simulink model "EKF_SIL_02_newdelIps"  (R2015a)
settings: Solver=ode45  StartTime=0.0  StopTime=totalSimulationTime  RelTol=1e-3
model workspace: external: MATLAB File Init_Model_02_Simulink_SIL1.m (data not in the file)
values from neighbouring files (symbols this model uses):
  Cov_nu = [0.005 0 0 0 ... (first row only)    [InitOOSM.m]    (also in InitSIL.m; Init_Model_02_Simulink.m; Init_Model_02_Simulink_SIL1.m)
  Cov_r = [0.003 0 0 ... (first row only)    [InitOOSM.m]    (also in InitSIL.m; Init_Model_02_Simulink.m; Init_Model_02_Simulink_SIL1.m)
  e_force_x = 0    [InitOOSM.m]    (also in InitSIL.m; Init_Model_02_Simulink.m; Init_Model_02_Simulink_SIL1.m)
  e_force_y = 0    [InitOOSM.m]    (also in InitSIL.m; Init_Model_02_Simulink.m; Init_Model_02_Simulink_SIL1.m)
  e_force_z = 0    [InitOOSM.m]    (also in InitSIL.m; Init_Model_02_Simulink.m; Init_Model_02_Simulink_SIL1.m)
  ieps = [-0.7071;0;0;0.7071]    [InitOOSM.m]    (also in InitSIL.m; Init_Model_02_Simulink.m = [-0.7071; 0; 0; 0.7071]; Init_Model_02_Simulink_SIL1.m)
  ita = [0.5;0.5;0.5;0.5]    [InitOOSM.m]    (also in InitSIL.m; Init_Model_02_Simulink.m = [0.5; 0.5; 0.5; 0.5]; Init_Model_02_Simulink_SIL1.m)
  n = 0.00    (= 0)    [InitOOSM.m]    (also in InitSIL.m; Init_Model_02_Simulink.m; Init_Model_02_Simulink_SIL1.m)
  P_0 = 0.5*eye(18,18)    [InitOOSM.m]    (also in InitSIL.m = 0.05*eye(12,12); Init_Model_02_Simulink.m = 0.005*eye(12,12); Init_Model_02_Simulink_SIL1.m = 0.005*eye(12,12))
  p_x = 0.75    [InitOOSM.m]    (also in InitSIL.m; Init_Model_02_Simulink.m; Init_Model_02_Simulink_SIL1.m)
  p_y = 0.125    [InitOOSM.m]    (also in InitSIL.m; Init_Model_02_Simulink.m; Init_Model_02_Simulink_SIL1.m)
  p_z = -0.8    [InitOOSM.m]    (also in InitSIL.m; Init_Model_02_Simulink.m; Init_Model_02_Simulink_SIL1.m)
  parameter_gravitation = 3.986005E+14    (= 398600500000000)    [InitOOSM.m]    (also in InitSIL.m; Init_Model_02_Simulink.m; Init_Model_02_Simulink_SIL1.m)
  rho = [0.04;0;0.3]    [InitOOSM.m]    (also in InitSIL.m; Init_Model_02_Simulink.m = [0.04; 0; 0.3]; Init_Model_02_Simulink_SIL1.m)
  rho_c = [-0.00017;   -0.9780;   -0.1854]    [InitOOSM.m]    (also in InitSIL.m = [0.00036;   -0.9865;   -0.1854]; Init_Model_02_Simulink.m = [0.00036; -0.9865; -0.1854]; Init_Model_02_Simulink_SIL1.m = [0.00036;   -0.9865;   -0.1854])
  sig_f = 2E-6    (= 2e-06)    [InitOOSM.m]    (also in InitSIL.m; Init_Model_02_Simulink.m; Init_Model_02_Simulink_SIL1.m)
  sig_tau = 2.5E-5    (= 2.5e-05)    [InitOOSM.m]    (also in InitSIL.m; Init_Model_02_Simulink.m; Init_Model_02_Simulink_SIL1.m)
  t_delta = 0.2    [InitOOSM.m]    (also in InitSIL.m; Init_Model_02_Simulink.m; Init_Model_02_Simulink_SIL1.m)
  t_Kalman = 0.01    [InitOOSM.m]    (also in InitSIL.m; Init_Model_02_Simulink.m; Init_Model_02_Simulink_SIL1.m)
  t_RobotSense = 0.05    [InitOOSM.m]    (also in InitSIL.m; Init_Model_02_Simulink.m; Init_Model_02_Simulink_SIL1.m)
  tau_1 = 0    [InitOOSM.m]    (also in InitSIL.m; Init_Model_02_Simulink.m; Init_Model_02_Simulink_SIL1.m)
  tau_2 = 0    [InitOOSM.m]    (also in InitSIL.m; Init_Model_02_Simulink.m; Init_Model_02_Simulink_SIL1.m)
  tau_3 = 0    [InitOOSM.m]    (also in InitSIL.m; Init_Model_02_Simulink.m; Init_Model_02_Simulink_SIL1.m)
  U_n_d = Simulink.Signal    [InitOOSM.m]    (also in InitSIL.m; Init_Model_02_Simulink.m; Init_Model_02_Simulink_SIL1.m)
  X_a_0 = [0; 0; 0; 1; 0; 0; 0; 0; 0; 0; 0; 0; 0;0;0;0;0;0;0;1]    [InitOOSM.m]    (also in InitSIL.m = [0; 0; 0; 1; 0; 0; 0; 0; 0; 0; 0; 0; 0]; Init_Model_02_Simulink.m = [0;0;0;0.707000000000000;0.707000000000000;0.200000000000000; Init_Model_02_Simulink_SIL1.m = [0;0;0.707;0.707;0.2;-0.02;0.0001;0.02;-1.80;0.50;-0.05;0.00)
libraries: simulink x5, dspmtrx3 x2, aerolibtransform2 x2, visionsinks x1
(part 1 of 4)
settings Model: PauseTimes=0  NumberOfSteps=10  SnapshotBufferSize=1  CovSFcnEnable=off  Creator=Iseberg  LastModifiedBy=Ana
settings DebuggingCC: SolverPrmCheckMsg=warning

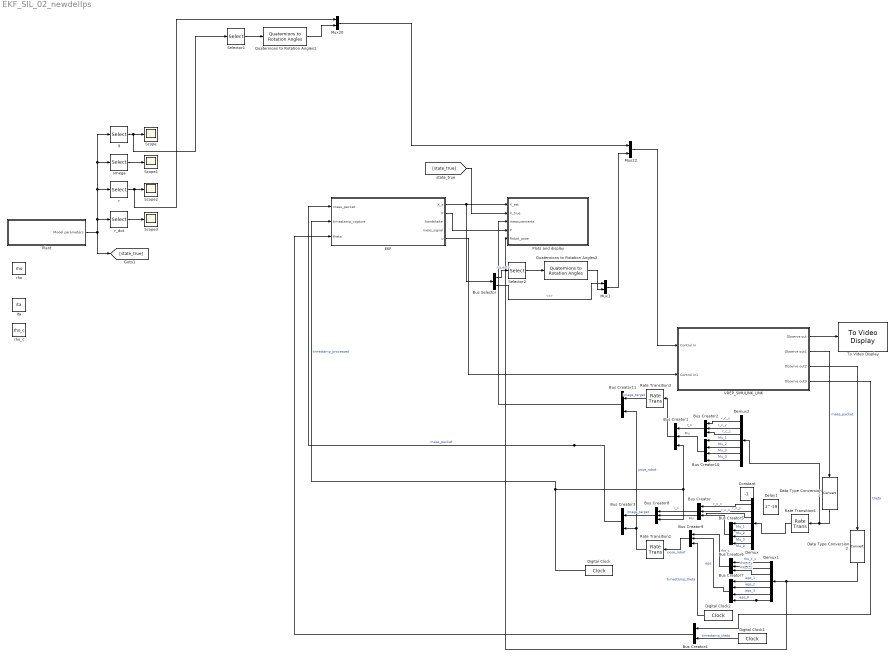
== system EKF_SIL_02_newdelIps ==
  Bus Creator{,1..2,6,8..9} (6 alike) : BusCreator  Inputs=3
  Bus Creator10 : BusCreator
  Bus Creator11 : BusCreator  Inputs=2
  Bus Creator3 : BusCreator  Inputs=2
  Bus Creator4 : BusCreator  Inputs=2
  Bus Creator5 : BusCreator
  Bus Creator7 : BusCreator
  Bus Selector : BusSelector  OutputSignals=q_est,r
  Constant : Constant  Value=-1
  Data Type Conversion1 : DataTypeConversion
  Data Type Conversion2 : DataTypeConversion
  Delay1 : Delay  DelayLength=19  InitialCondition=0  SampleTime=t_Kalman
  Demux : Demux  Outputs=7
  Demux1 : Demux  Outputs=7
  Demux2 : Demux  Outputs=7
  Digital Clock : DigitalClock  SampleTime=t_delta
  Digital Clock1 : DigitalClock  SampleTime=t_Kalman
  Digital Clock2 : DigitalClock  SampleTime=t_RobotSense
  EKF : Subsystem  TreatAsAtomicUnit=on  SystemSampleTime=t_Kalman
  Mux1 : Mux  Inputs=2
  Mux20 : Mux  Inputs=2
  Mux22 : Mux  Inputs=2
  Plant : Subsystem
  Plots and display : Subsystem
  Quaternions to Rotation Angles1 : aerolibtransform2/Quaternions to Rotation Angles  rotationOrder=XYZ
  Quaternions to Rotation Angles2 : aerolibtransform2/Quaternions to Rotation Angles  rotationOrder=XYZ
  Rate Transition2 : RateTransition  OutPortSampleTime=t_RobotSense
  Rate Transition3 : RateTransition  OutPortSampleTime=t_delta
  Rate Transition4 : RateTransition  OutPortSampleTime=t_delta
  Scope{,1..3} (4 alike) : Scope
      Scope settings: ShowLegends=on  YMin=-1  YMax=1  MaxDataPoints=100000
      Scope1 settings: ShowLegends=on  TimeRange=40
      Scope2 settings: ShowLegends=on  SaveName=ScopeData2
      Scope3 settings: ShowLegends=on  SaveName=ScopeData3
  Selector1 : Selector  InputPortWidth=4  Indices=[4 1 2 3]
  Selector2 : Selector  InputPortWidth=4  Indices=[4 1 2 3]
  To Video Display : visionsinks/To Video Display  windowSizeMode=True size (1:1)  openAtMdlStart=on  fullScreen=off  videoWindowX=32768  videoWindowY=32766  saveWindowSize=off  videoWindowWidth=512  videoWindowHeight=512  inputColorFormat=RGB  inputType=Obsolete  imagePorts=One multidimensional signal  OutputDevice=On-screen video monitor  dataOrg=Column-major  isWindowOpen=on
  VREP_SIMULINK_LINK : Subsystem  SystemSampleTime=t_delta  mask{ObjectsInScene=DefaultCamera, m_ControlObjects={ 'Client_Real','BaseFrame';'Client_Est','BaseFrame';'UR5_joint1','Joint';'UR5_joint2','Joint';'UR5_joint3','Joint';}, m_InitialControllablePose={[X_a_0_sim.X_a_0_Model_02(9:11);X_a_0_sim.eulerAngles_X_a_0'];zeros(6,1)}, m_ObserveObjects={'Vision_sensor','Image',''; 'apriltag','Pose','Vision_sensor';  'BaseFrame','Pose','Vision_sensor';'UR5_joint1','Joint','';'UR5_joint2','Joint','';'UR5_joint3','Joint','';'UR5_joint4','Joint','';'UR5_joint5','Joint','';'UR5_joint6','Joint',''}, sceneFileName=scene_OOSM.ttt, OutPortSampleTime=0.05}
      mask prompts: ObjectsInScene "Objects present in scene:"; m_ControlObjects "Control Objects:"; m_InitialControllablePose "Initial Pose:"; m_ObserveObjects "Observing Objects:"; sceneFileName "Scene filename:"; OutPortSampleTime "VREP Sample time [s]"
      mask TypeOptions ObjectsInScene: DefaultCamera | DefaultXViewCamera | DefaultYViewCamera | DefaultZViewCamera | XYZCameraProxy | DefaultNXViewCamera | DefaultNYViewCamera | DefaultNZViewCamera | DefaultLightA | DefaultLightB | DefaultLightC | DefaultLightD | UR5_link1_visible | UR5_joint1 | UR5_link2 | UR5_link2_visible | UR5_joint2 | UR5_link3 | UR5_link3_visible | UR5_joint3 | UR5_link4 | UR5_link4_visible | UR5_joint4 | UR5_link5 | UR5_link5_visible | UR5_joint5 | UR5_link6 | UR5_joint6 | UR5_link7 | UR5_link7_visible | UR5_connection | UR5_link6_visible | DH_J2 | DH_J1 | DH_J3 | DH_J4 | DH_J5 | DH_J6 | DH_tool | BaseFrame | UR5_target | Vision_sensor | apriltag | Client_Est | Client_Real | Grasping_real | Grasping_est | BaseFrame_Est | ReferenceFrame_shape | Origin | Servicer_UR5
      mask TypeOptions m_ControlObjects: VREP_SIMULINK_SYS_OBJ/m_ControlObjects
      mask TypeOptions m_InitialControllablePose: VREP_SIMULINK_SYS_OBJ/m_InitialControllablePose
      mask TypeOptions m_ObserveObjects: VREP_SIMULINK_SYS_OBJ/m_ObserveObjects
      mask TypeOptions sceneFileName: VREP_SIMULINK_SYS_OBJ/sceneFileName
      mask TypeOptions OutPortSampleTime: Rate Transition/OutPortSampleTime | Rate Transition1/OutPortSampleTime
      mask DialogControl Control1 Prompt: V-REP Simulink LINK block settings
      mask DialogControl Container8 Prompt: V-REP settings
      mask Display:
      | image('vrepProEdu.png')
      | port_label('input',1,'Control in');
      | port_label('output',1,'Observe out');
  ita : Constant  Value=ita
  omega : Selector  NumberOfDimensions=2  InputPortWidth=3  IndexOptions=Index vector (dialog),Index vector (dialog)  Indices=[5 6 7],1  OutputSizes=1,1
  q : Selector  NumberOfDimensions=2  InputPortWidth=3  IndexOptions=Index vector (dialog),Index vector (dialog)  Indices=[1 2 3 4],1  OutputSizes=1,1
  r : Selector  NumberOfDimensions=2  InputPortWidth=3  IndexOptions=Index vector (dialog),Index vector (dialog)  Indices=[8 9 10],1  OutputSizes=1,1
  r_dot : Selector  NumberOfDimensions=2  InputPortWidth=3  IndexOptions=Index vector (dialog),Index vector (dialog)  Indices=[11 12 13],1  OutputSizes=1,1
  "rho " : Constant  Value=rho
  rho_c : Constant  Value=rho_c
  wires:
  omega/1 -> Scope1/1
  r_dot/1 -> Scope3/1
  Plant/1(Model parameters) -> [state_true], omega/1, q/1, r/1, r_dot/1
  q/1 -> Selector1/1, Scope/1
  r/1 -> Mux20/1, Scope2/1
  [state_true] -> Plots and display/2(X_true)
  EKF/2(P) -> Plots and display/4(P)
  EKF/1(X_a) -> Bus Selector/1, Plots and display/1(X_est)
  Mux22/1 -> VREP_SIMULINK_LINK/1(Control In)
  Selector1/1 -> Quaternions to Rotation Angles1/1
  Quaternions to Rotation Angles1/1 -> Mux20/2
  Bus Selector/1 -> Selector2/1  "<q_est>"
  Bus Selector/2 -> Mux1/1  "<r>"
  Quaternions to Rotation Angles2/1 -> Mux1/2
  Mux1/1 -> Mux22/2
  Mux20/1 -> Mux22/1
  VREP_SIMULINK_LINK/1(Observe out) -> To Video Display/1
  Selector2/1 -> Quaternions to Rotation Angles2/1
  VREP_SIMULINK_LINK/2(Observe out1) -> Data Type Conversion1/1  "meas_packet"
  Digital Clock/1 -> EKF/2("timestamp_capture "), Bus Creator1/3, Bus Creator8/3  "timestamp_processed"
  Demux/4 -> Bus Creator5/1  "Mu_1"
  Demux/5 -> Bus Creator5/2  "Mu_2"
  Demux/6 -> Bus Creator5/3  "Mu_3"
  Demux/7 -> Bus Creator5/4  "Mu_0"
  Demux/1 -> Bus Creator/1  "r_c_x"
  Demux/2 -> Bus Creator/2  "r_c_y"
  Demux/3 -> Bus Creator/3  "r_c_z"
  Bus Creator/1 -> Bus Creator8/1  "r_c"
  Bus Creator3/1 -> EKF/1(meas_packet)  "meas_packet"
  VREP_SIMULINK_LINK/3(Observe out2) -> Data Type Conversion2/1
  Demux1/4 -> Bus Creator7/1  "ieps_1"
  Demux1/5 -> Bus Creator7/2  "ieps_2"
  Demux1/6 -> Bus Creator7/3  "ieps_3"
  Demux1/7 -> Bus Creator7/4  "ieps_0"
  Demux1/2 -> Bus Creator6/2  "rho_c_y"
  Demux1/1 -> Bus Creator6/1  "rho_c_x"
  Demux1/3 -> Bus Creator6/3  "rho_c_z"
  Bus Creator6/1 -> Bus Creator9/1  "rho_c"
  Bus Creator7/1 -> Bus Creator9/2  "ieps"
  Bus Creator4/1 -> EKF/3(theta)
  VREP_SIMULINK_LINK/4(Observe out3) -> Bus Creator4/1  "theta"
  Digital Clock1/1 -> Bus Creator4/2  "timestamp_theta"
  Bus Creator5/1 -> Bus Creator8/2  "Mu"
  EKF/5(u) -> VREP_SIMULINK_LINK/2(Control In1)
  Bus Creator9/1 -> Rate Transition2/1  "pose_robot"
  Digital Clock2/1 -> Bus Creator9/3  "timestamp_theta"
  Rate Transition2/1 -> Bus Creator11/2, Bus Creator3/2  "pose_robot"
  Data Type Conversion2/1 -> Plots and display/5("Robot_pose "), Demux1/1
  Demux2/4 -> Bus Creator10/1  "Mu_1"
  Demux2/5 -> Bus Creator10/2  "Mu_2"
  Demux2/6 -> Bus Creator10/3  "Mu_3"
  Demux2/1 -> Bus Creator2/1  "r_c_x"
  Demux2/2 -> Bus Creator2/2  "r_c_y"
  Demux2/3 -> Bus Creator2/3  "r_c_z"
  Bus Creator2/1 -> Bus Creator1/1  "r_c"
  Bus Creator10/1 -> Bus Creator1/2  "Mu"
  Demux2/7 -> Bus Creator10/4  "Mu_0"
  Bus Creator1/1 -> Rate Transition3/1
  Rate Transition3/1 -> Bus Creator11/1  "image_target"
  Bus Creator11/1 -> Plots and display/3(measurements)
  Data Type Conversion1/1 -> Rate Transition4/1, Demux2/1
  Bus Creator8/1 -> Bus Creator3/1  "image_target"
  Rate Transition4/1 -> Demux/1

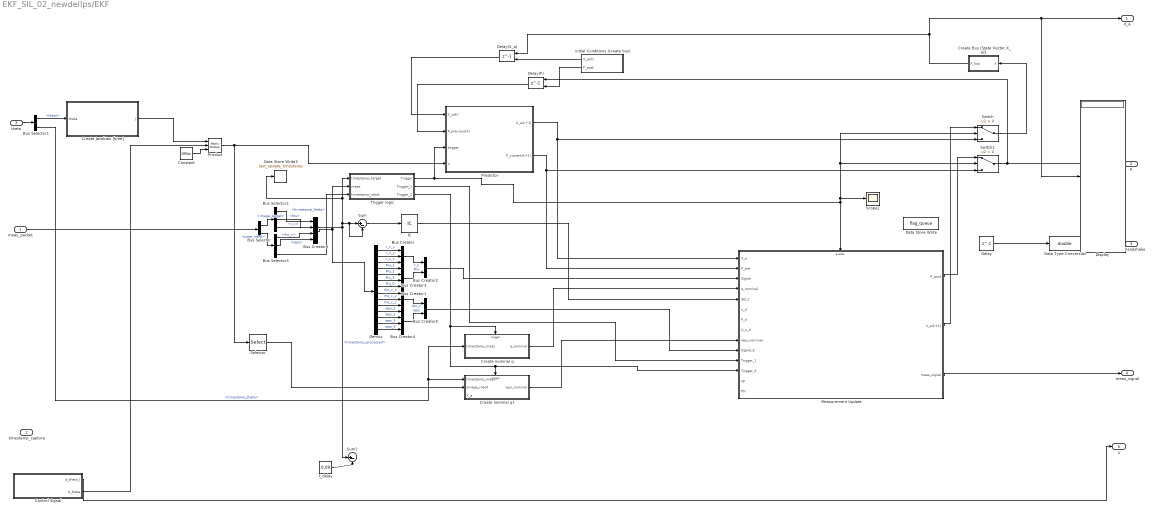
== system EKF_SIL_02_newdelIps/EKF ==
  meas_packet : Inport
  "timestamp_capture " : Inport  Port=2
  theta : Inport  Port=3
  Bus Creator : BusCreator  Inputs=3
  Bus Creator1 : BusCreator
  Bus Creator2 : BusCreator  Inputs=2
  Bus Creator3 : BusCreator  Inputs=3
  Bus Creator4 : BusCreator
  Bus Creator5 : BusCreator  Inputs=2
  Bus Creator6 : BusCreator
  Bus Selector : BusSelector  OutputSignals=image_target,pose_robot
  Bus Selector1 : BusSelector  OutputSignals=theta,timestamp_theta
  Bus Selector2 : BusSelector  OutputSignals=r_c,Mu,timestamp_processed
  Bus Selector3 : BusSelector  OutputSignals=rho_c,ieps,timestamp_theta
  Constant : Constant  Value=180/pi
  Control Signal : Subsystem
  Create Bus [State Vector,X_a]1 : Subsystem
  Create Jacobian [b/ee] : Subsystem
  Create nominal q : Subsystem  TreatAsAtomicUnit=on
  Create nominal q1 : Subsystem  TreatAsAtomicUnit=on
  Data Store Write : DataStoreWrite  DataStoreName=flag_queue
  Data Store Write3 : DataStoreWrite  DataStoreName=last_update_timestamp
  Data Type Conversion : DataTypeConversion  OutDataTypeStr=double  LockScale=on
  Delay : Delay  DelayLength=1  InitialCondition=0
  Delay(P) : Delay  DelayLength=1  InitialConditionSource=Input port  InitialCondition=0  SampleTime=t_Kalman
      settings: InputPortMap=u0,p4
  Delay(X_a) : Delay  DelayLength=1  InitialConditionSource=Input port  InitialCondition=0  SampleTime=t_Kalman
      settings: InputPortMap=u0,p4
  Demux : Demux  Outputs=14
  Display : Display
  IC : InitialCondition  Value=0
  Initial Conditions (create bus) : Subsystem
  Measurement Update : Subsystem  TreatAsAtomicUnit=on
  Predictor : Subsystem  TreatAsAtomicUnit=on  SystemSampleTime=t_Kalman
  Product : Product  Inputs=3  Multiplication=Matrix(*)
  Scope2 : Scope
      settings: YMin=0  YMax=1  SaveName=ScopeData5
  Selector : Selector  InputPortWidth=6  Indices=[4:6]
  Sum : Sum  Inputs=|+-
  Sum1 : Sum  Inputs=|+-
  Switch : Switch  Criteria=u2 > Threshold
  Switch1 : Switch  Criteria=u2 > Threshold
  Trigger logic : Subsystem
  "t_delay " : Constant  Value=0.09
  X_a : Outport
  P : Outport  Port=2
  handshake : Outport  Port=3
  meas_signal : Outport  Port=4
  u : Outport  Port=5
  wires:
  meas_packet/1 -> Bus Selector/1
  Predictor/2(P_current(k+1)) -> Switch1/3, Measurement Update/2(P_pre)
  Measurement Update/1(P_post) -> Switch1/1
  Initial Conditions (create bus)/2("P_post ") -> Delay(P)/2
  Switch1/1 -> Delay(P)/1, P/1
  Delay(P)/1 -> Predictor/2(P_previous(k))
  Demux/1 -> Bus Creator/1  "r_c_x"
  Demux/2 -> Bus Creator/2  "r_c_y"
  Demux/3 -> Bus Creator/3  "r_c_z"
  Demux/4 -> Bus Creator1/1  "Mu_1"
  Demux/5 -> Bus Creator1/2  "Mu_2"
  Demux/6 -> Bus Creator1/3  "Mu_3"
  Demux/7 -> Bus Creator1/4  "Mu_0"
  Bus Creator/1 -> Bus Creator2/1  "r_c"
  Bus Creator1/1 -> Bus Creator2/2  "Mu"
  Initial Conditions (create bus)/1("X_a(0) ") -> Delay(X_a)/2
  Create nominal q/1(q_nominal) -> Measurement Update/4("q_nominal ")
  Bus Creator2/1 -> Measurement Update/3(Signal)
  Sum/1 -> IC/1
  IC/1 -> Measurement Update/5(del_t)
  Delay/1 -> Data Type Conversion/1
  Data Type Conversion/1 -> handshake/1
  Predictor/1(X_a(k+1)) -> Switch/3, Measurement Update/1(X_a)
  Measurement Update/3(meas_signal) -> meas_signal/1
  Bus Selector2/3 -> Trigger logic/1(timestamp_target), Data Store Write3/1, Sum/2, Sum/1, Sum1/1  "<timestamp_processed>"
  Bus Creator6/1 -> Demux/1, Trigger logic/2(meas)
  theta/1 -> Bus Selector1/1
  Trigger logic/1("Trigger ") -> Measurement Update/Enable, Scope2/1, Switch1/2, Switch/2, Predictor/3(trigger)
  Product/1 -> Selector/1, Predictor/4(V)
  Create Jacobian [b/ee]/1(J) -> Product/1
  Bus Selector1/1 -> Create Jacobian [b/ee]/1(theta)  "<theta>"
  Bus Selector1/2 -> Create nominal q/1(timestamp_meas), Create nominal q1/1(timestamp_meas)  "<timestamp_theta>"
  Selector/1 -> Create nominal q1/2(omega_robot)
  Measurement Update/2(X_a(k+1)) -> Switch/1
  Create nominal q1/1(ieps_nominal) -> Measurement Update/9(ieps_nominal)
  Constant/1 -> Product/3
  Control Signal/1(d_theta_l) -> u/1
  Demux/8 -> Bus Creator3/1  "rho_c_x"
  Demux/9 -> Bus Creator3/2  "rho_c_y"
  Demux/10 -> Bus Creator3/3  "rho_c_z"
  Demux/11 -> Bus Creator4/1  "ieps_1"
  Demux/12 -> Bus Creator4/2  "ieps_2"
  Demux/13 -> Bus Creator4/3  "ieps_3"
  Demux/14 -> Bus Creator4/4  "ieps_0"
  Bus Creator3/1 -> Bus Creator5/1  "rho_c"
  Bus Creator4/1 -> Bus Creator5/2  "ieps"
  Bus Creator5/1 -> Measurement Update/10(Signal_b)
  Control Signal/2(d_theta) -> Product/2
  Bus Selector/1 -> Bus Selector2/1  "<image_target>"
  Bus Selector/2 -> Bus Selector3/1  "<pose_robot>"
  Bus Selector2/1 -> Bus Creator6/1  "<r_c>"
  Bus Selector2/2 -> Bus Creator6/2  "<Mu>"
  Bus Selector3/2 -> Bus Creator6/4  "<ieps>"
  Bus Selector3/3 -> Trigger logic/3(timestamp_robot)  "<timestamp_theta>"
  Bus Selector3/1 -> Bus Creator6/3  "<rho_c>"
  Trigger logic/2("Trigger_1 ") -> Measurement Update/11(Trigger_1)
  Trigger logic/3("Trigger_2 ") -> Measurement Update/12(Trigger_2), Create nominal q1/Trigger, Create nominal q/Trigger
  Delay(X_a)/1 -> Predictor/1(X_a(K))
  "t_delay "/1 -> Sum1/2
  Create Bus [State Vector,X_a]1/1(X_bus) -> Delay(X_a)/1, Display/1, X_a/1
  Switch/1 -> Create Bus [State Vector,X_a]1/1(X)

== system EKF_SIL_02_newdelIps/Plant ==
  Dynamic Model (Differential equations) : Subsystem
  Initial Conditions (create bus) : Subsystem
  Integrator : Integrator  InitialConditionSource=external
  Selector2 : Selector  NumberOfDimensions=2  InputPortWidth=3  IndexOptions=Index vector (dialog),Index vector (dialog)  Indices=[1:13],1  OutputSizes=1,1
  Model parameters : Outport
  wires:
  Integrator/1 -> Model parameters/1, Dynamic Model (Differential equations)/1(X_a(t))
  Initial Conditions (create bus)/1("X_a(0) ") -> Selector2/1
  Selector2/1 -> Integrator/2
  Dynamic Model (Differential equations)/1(X_a(t+1)) -> Integrator/1

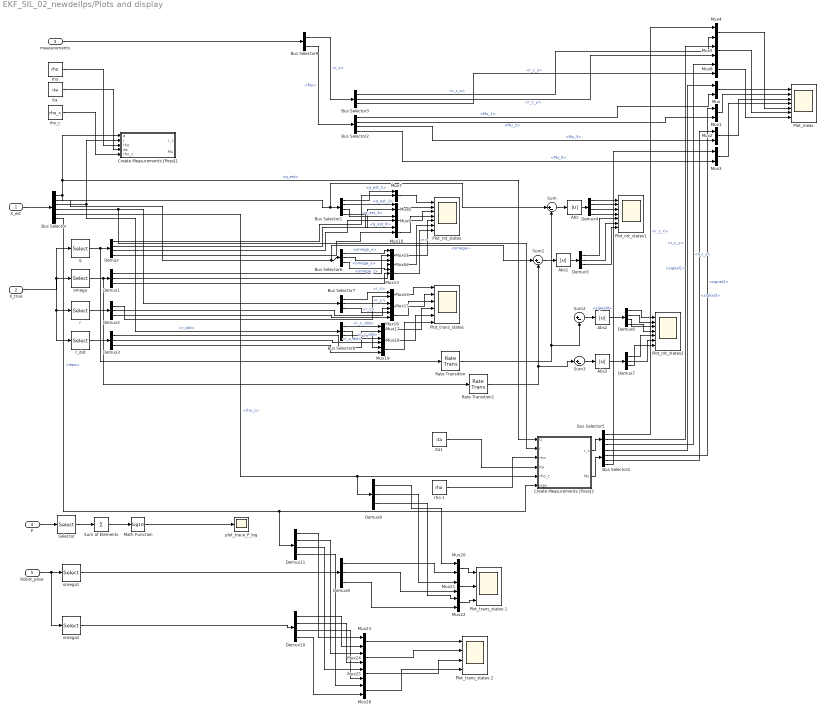
== system EKF_SIL_02_newdelIps/Plots and display ==
  X_est : Inport
  X_true : Inport  Port=2
  measurements : Inport  Port=3
  P : Inport  Port=4
  "Robot_pose " : Inport  Port=5
  Abs{,1..3} (4 alike) : Abs
  Bus Selector : BusSelector  OutputSignals=q_est,omega,r,r_dot,rho_c,ieps
  Bus Selector1 : BusSelector  OutputSignals=q_est_1,q_est_2,q_est_3,q_est_0
  Bus Selector2 : BusSelector  OutputSignals=Mu_1,Mu_2,Mu_3,Mu_0
  Bus Selector3 : BusSelector  OutputSignals=r_c_x,r_c_y,r_c_z
  Bus Selector4 : BusSelector  OutputSignals=signal1,signal2,signal3,signal4
  Bus Selector5 : BusSelector  OutputSignals=r_c_x,r_c_y,r_c_z
  Bus Selector6 : BusSelector  OutputSignals=omega_x,omega_y,omega_z
  Bus Selector7 : BusSelector  OutputSignals=r_x,r_y,r_z
  Bus Selector8 : BusSelector  OutputSignals=r_x_dot,r_y_dot,r_z_dot
  Bus Selector9 : BusSelector  OutputSignals=image_target.r_c,image_target.Mu
  Create Measurements [Pose]1 : Subsystem
  Create Measurements [Pose]2 : Subsystem
  Demux{,4,6,10..11} (5 alike) : Demux
  Demux{1..3,5,7..9} (7 alike) : Demux  Outputs=3
  Math Function : Math  Operator=log10  SaturateOnIntegerOverflow=on
  Mux{,1..6,14..26} (20 alike) : Mux  Inputs=2
  Mux{7..13} (7 alike) : Mux  Inputs=3
  "Plot_meas " : Scope  NumInputPorts=7
      settings: ShowLegends=on  TimeRange=100  YMin=-0.75~-1~-0.15~-0.4~-1.5~-1~0.9  YMax=1~1~0.2~0.4~0.25~-0.1~1.7  SaveName=ScopeData9
  Plot_rot_states : Scope  NumInputPorts=7
      settings: ShowLegends=on  TimeRange=30  YMin=0~0~0~0~0~-0.02~0  YMax=0.8~0.6~0.8~0.8~0.3~0~0.035  SaveName=ScopeData24
  Plot_rot_states1 : Scope  NumInputPorts=7
      settings: ShowLegends=on  TimeRange=100  YMin=-1~-1~-1~-0.75~0~-0.4~-1  YMax=1~1~1~1~1~0.4~1  SaveName=ScopeData14
  Plot_rot_states2 : Scope  NumInputPorts=7
      settings: ShowLegends=on  TimeRange=100  YMin=-3.46945e-18~-3.46945e-18~-1.38778e-17~-2.77556e-17~0.05~1.38778e-17~5.55112e-17  YMax=0.1~0.14~0.175~0.35~0.35~0.25~0.9  SaveName=ScopeData15
  "Plot_trans_states " : Scope  NumInputPorts=6
      settings: ShowLegends=on  TimeRange=100  YMin=-0.7~-1.805~0.493~-0.05~-0.0006~-0.0035  YMax=0.1~-1.798~0.504~-0.0375~0.0002~0.0005  SaveName=ScopeData11
  Plot_trans_states 1 : Scope  NumInputPorts=3
      settings: ShowLegends=on  TimeRange=50  YMin=-0.0025~-1~-0.19  YMax=0.0275~0~0  SaveName=ScopeData7
  Plot_trans_states 2 : Scope  NumInputPorts=4
      settings: ShowLegends=on  TimeRange=30  YMin=-0.7075~-0.2~-0.002~0.706925  YMax=-0.6825~0.025~0.0005~0.7071  SaveName=ScopeData8
  Rate Transition : RateTransition
  Rate Transition1 : RateTransition
  Selector : Selector  NumberOfDimensions=2  InputPortWidth=3  IndexOptions=Index vector (dialog),Index vector (dialog)  Indices=[1:12],[1:12]  OutputSizes=1,1
  Sum{,1..3} (4 alike) : Sum  Inputs=|+-
  Sum of Elements : Sum  Inputs=+
  ita : Constant  Value=ita
  ita1 : Constant  Value=ita
  omega : Selector  NumberOfDimensions=2  InputPortWidth=3  IndexOptions=Index vector (dialog),Index vector (dialog)  Indices=[5 6 7],1  OutputSizes=1,1
  omega1 : Selector  InputPortWidth=7  Indices=[1:3]
  omega2 : Selector  InputPortWidth=7  Indices=[4:7]
  plot_trace_P_log : Scope
      settings: ShowLegends=on  TimeRange=100  YMin=-1.3  YMax=0.7  SaveName=ScopeData4
  q : Selector  NumberOfDimensions=2  InputPortWidth=3  IndexOptions=Index vector (dialog),Index vector (dialog)  Indices=[1 2 3 4],1  OutputSizes=1,1
  r : Selector  NumberOfDimensions=2  InputPortWidth=3  IndexOptions=Index vector (dialog),Index vector (dialog)  Indices=[8 9 10],1  OutputSizes=1,1
  r_dot : Selector  NumberOfDimensions=2  InputPortWidth=3  IndexOptions=Index vector (dialog),Index vector (dialog)  Indices=[11 12 13],1  OutputSizes=1,1
  "rho " : Constant  Value=rho
  rho 1 : Constant  Value=rho
  rho_c : Constant  Value=rho_c
  wires:
  Bus Selector/1 -> Sum/1, Bus Selector1/1, Create Measurements [Pose]2/1(q), Create Measurements [Pose]1/1(q)  "<q_est>"
  Bus Selector/3 -> Create Measurements [Pose]2/2(r), Bus Selector7/1, Create Measurements [Pose]1/2(r)  "<r>"
  Bus Selector1/1 -> Mux7/1  "<q_est_1>"
  Mux7/1 -> Plot_rot_states/1
  Demux/1 -> Mux7/2
  Bus Selector1/2 -> Mux8/1  "<q_est_2>"
  Demux/2 -> Mux8/2
  Bus Selector1/3 -> Mux9/1  "<q_est_3>"
  Demux/3 -> Mux9/2
  Bus Selector1/4 -> Mux10/1  "<q_est_0>"
  Demux/4 -> Mux10/2
  Mux8/1 -> Plot_rot_states/2
  Mux9/1 -> Plot_rot_states/3
  Mux10/1 -> Plot_rot_states/4
  Bus Selector/2 -> Sum1/1, Bus Selector6/1  "<omega>"
  Bus Selector6/1 -> Mux11/1  "<omega_x>"
  Demux1/1 -> Mux11/2
  Bus Selector6/2 -> Mux12/1  "<omega_y>"
  Demux1/2 -> Mux12/2
  Bus Selector6/3 -> Mux13/1  "<omega_z>"
  Demux1/3 -> Mux13/2
  Mux11/1 -> Plot_rot_states/5
  Mux12/1 -> Plot_rot_states/6
  Mux13/1 -> Plot_rot_states/7
  Bus Selector7/1 -> Mux14/1  "<r_x>"
  Demux2/1 -> Mux14/2
  Bus Selector7/2 -> Mux15/1  "<r_y>"
  Demux2/2 -> Mux15/2
  Bus Selector7/3 -> Mux16/1  "<r_z>"
  Demux2/3 -> Mux16/2
  Mux14/1 -> "Plot_trans_states "/1
  Mux15/1 -> "Plot_trans_states "/2
  Mux16/1 -> "Plot_trans_states "/3
  Bus Selector/4 -> Bus Selector8/1  "<r_dot>"
  Bus Selector8/1 -> Mux17/1  "<r_x_dot>"
  Demux3/1 -> Mux17/2
  Bus Selector8/2 -> Mux18/1  "<r_y_dot>"
  Demux3/2 -> Mux18/2
  Bus Selector8/3 -> Mux19/1  "<r_z_dot>"
  Demux3/3 -> Mux19/2
  Mux17/1 -> "Plot_trans_states "/4
  Mux18/1 -> "Plot_trans_states "/5
  Mux19/1 -> "Plot_trans_states "/6
  X_est/1 -> Bus Selector/1
  X_true/1 -> r_dot/1, r/1, omega/1, q/1
  q/1 -> Rate Transition/1, Demux/1
  omega/1 -> Rate Transition1/1, Demux1/1
  r_dot/1 -> Demux3/1
  r/1 -> Demux2/1
  Bus Selector2/1 -> Mux/2  "<Mu_1>"
  Bus Selector2/2 -> Mux1/2  "<Mu_2>"
  Bus Selector2/3 -> Mux2/2  "<Mu_3>"
  Bus Selector4/4 -> Mux3/1  "<signal4>"
  Bus Selector2/4 -> Mux3/2  "<Mu_0>"
  Mux/1 -> "Plot_meas "/1
  Mux1/1 -> "Plot_meas "/2
  Mux2/1 -> "Plot_meas "/3
  Mux3/1 -> "Plot_meas "/4
  Bus Selector3/1 -> Mux4/2  "<r_c_x>"
  Bus Selector3/2 -> Mux5/2  "<r_c_y>"
  Bus Selector3/3 -> Mux6/2  "<r_c_z>"
  Mux4/1 -> "Plot_meas "/5
  Mux5/1 -> "Plot_meas "/6
  Mux6/1 -> "Plot_meas "/7
  "rho "/1 -> Create Measurements [Pose]1/3(rho)
  ita/1 -> Create Measurements [Pose]1/4(ita)
  rho_c/1 -> Create Measurements [Pose]1/5("rho_c ")
  measurements/1 -> Bus Selector9/1
  Bus Selector9/1 -> Bus Selector3/1  "<r_c>"
  Bus Selector9/2 -> Bus Selector2/1  "<Mu>"
  P/1 -> Selector/1
  Selector/1 -> Sum of Elements/1
  Sum of Elements/1 -> Math Function/1
  Math Function/1 -> plot_trace_P_log/1
  Rate Transition/1 -> Sum2/2, Sum/2
  Sum/1 -> Abs/1
  Abs/1 -> Demux4/1
  Demux4/1 -> Plot_rot_states1/1
  Demux4/2 -> Plot_rot_states1/2
  Demux4/3 -> Plot_rot_states1/3
  Demux4/4 -> Plot_rot_states1/4
  Rate Transition1/1 -> Sum3/1, Sum1/2
  Sum1/1 -> Abs1/1
  Demux5/1 -> Plot_rot_states1/5
  Demux5/2 -> Plot_rot_states1/6
  Demux5/3 -> Plot_rot_states1/7
  Abs1/1 -> Demux5/1
  Sum2/1 -> Abs2/1
  Sum3/1 -> Abs3/1
  Abs2/1 -> Demux6/1
  Demux6/1 -> Plot_rot_states2/1
  Demux6/2 -> Plot_rot_states2/2
  Demux6/3 -> Plot_rot_states2/3
  Demux6/4 -> Plot_rot_states2/4
  Abs3/1 -> Demux7/1
  Demux7/1 -> Plot_rot_states2/5
  Demux7/2 -> Plot_rot_states2/6
  Demux7/3 -> Plot_rot_states2/7
  rho 1/1 -> Create Measurements [Pose]2/3(rho)
  ita1/1 -> Create Measurements [Pose]2/4(ita)
  Create Measurements [Pose]2/2(Mu) -> Bus Selector4/1
  Bus Selector4/3 -> Mux2/1  "<signal3>"
  Bus Selector4/2 -> Mux1/1  "<signal2>"
  Bus Selector4/1 -> Mux/1  "<signal1>"
  Create Measurements [Pose]2/1(r_c) -> Bus Selector5/1
  Bus Selector5/1 -> Mux4/1  "<r_c_x>"
  Bus Selector5/2 -> Mux5/1  "<r_c_y>"
  Bus Selector5/3 -> Mux6/1  "<r_c_z>"
  Bus Selector/5 -> Demux9/1, Create Measurements [Pose]2/5("rho_c ")  "<rho_c>"
  Bus Selector/6 -> Create Measurements [Pose]2/6(ieps), Demux11/1  "<ieps>"
  "Robot_pose "/1 -> omega2/1, omega1/1
  omega1/1 -> Demux8/1
  omega2/1 -> Demux10/1
  Demux8/1 -> Mux20/2
  Demux9/1 -> Mux20/1
  Mux20/1 -> Plot_trans_states 1/1
  Demux8/2 -> Mux21/2
  Demux9/3 -> Mux22/1
  Demux8/3 -> Mux22/2
  Mux21/1 -> Plot_trans_states 1/2
  Mux22/1 -> Plot_trans_states 1/3
  Demux11/1 -> Mux23/1
  Demux9/2 -> Mux21/1
  Demux10/1 -> Mux23/2
  Mux23/1 -> Plot_trans_states 2/1
  Demux10/2 -> Mux24/2
  Demux11/2 -> Mux24/1
  Demux10/3 -> Mux25/2
  Demux11/3 -> Mux25/1
  Demux10/4 -> Mux26/2
  Demux11/4 -> Mux26/1
  Mux24/1 -> Plot_trans_states 2/2
  Mux25/1 -> Plot_trans_states 2/3
  Mux26/1 -> Plot_trans_states 2/4

== system EKF_SIL_02_newdelIps/VREP_SIMULINK_LINK ==
  Control In : Inport
  Control In1 : Inport  Port=2
  Constant : Constant  Value=180/pi
  Mux : Mux  Inputs=6
  Product : Product
  Rate Transition{,1..5} (6 alike) : RateTransition  OutPortSampleTime=OutPortSampleTime
  Signal Specification : SignalSpecification  Dimensions=[12,1]
  Signal Specification1 : SignalSpecification  Dimensions=[3,1]
  VREP_SIMULINK_SYS_OBJ : MATLABSystem  System=SysObjVREP_1  ObjectsInScene={'DefaultCamera'; 'DefaultXViewCamera'; 'DefaultYViewCamera'; 'DefaultZViewCamera'; 'XYZCameraProxy'; 'DefaultNXViewCamera'; 'DefaultNYViewCamera'; 'DefaultNZViewCamera'; 'DefaultLightA'; 'DefaultLightB'; 'DefaultLightC'; 'DefaultLightD'; 'UR5'; 'UR5_link1_visible'; 'UR5_joint1'; 'UR5_link2'; 'UR5_link2_visible'; 'UR5_joint2'; 'UR5_link3'; 'UR5_link3_visible'; 'UR5_joint3'; 'UR5_link4'; 'UR5_link4_visible'; 'UR5_joint4'; 'UR5_link5'; 'UR5_link5_visible'; 'UR5_joint5'; 'UR5_link6'; 'UR5_joint6'; 'UR5_link7'; 'UR5_link7_visible'; 'UR5_connection'; 'UR5_link6_visible'; 'DH_J2'; 'DH_J1'; 'DH_J3'; 'DH_J4'; 'DH_J5'; 'DH_J6'; 'DH_tool'; 'BaseFrame'; 'UR5_target'; 'Vision_sensor'; 'apriltag'; 'Client_Est'; 'Client_Real'; 'Grasping_real'; 'Grasping_est'; 'BaseFrame_Est'; 'ReferenceFrame_shape'; 'Origin'}  sceneFileName=scene_OOSM.ttt  m_ControlObjects=m_ControlObjects  m_ObserveObjects=m_ObserveObjects  m_InitialControllablePose=m_InitialControllablePose  SimulateUsing=Interpreted execution
      mask Type: SysObjVREP_1
      mask Display:
      | disp('V-REP');
      | port_label('input',1,'Control(1)');
      | port_label('input',2,'Control(2)');
      | port_label('output',1,'Observe(1)');
      | port_label('output',2,'Observe(2)');
      | port_label('output',3,'Observe(3)');
      | port_label('output',4,'Observe(4)');
      | port_label('output',5,'Observe(5)');
      | port_label('output',6,'Observe(6)');
      | port_label('output',7,'Observe(7)');
      | port_label('output',8,'Observe(8)');
      | port_label('output',9,'Observe(9)');
  Observe out : Outport
  Observe out1 : Outport  Port=2
  Observe out2 : Outport  Port=3
  Observe out3 : Outport  Port=4
  wires:
  Control In/1 -> Signal Specification/1
  VREP_SIMULINK_SYS_OBJ/1 -> Rate Transition1/1
  Rate Transition/1 -> VREP_SIMULINK_SYS_OBJ/1
  Rate Transition1/1 -> Observe out/1
  Rate Transition2/1 -> Observe out1/1
  VREP_SIMULINK_SYS_OBJ/3 -> Rate Transition3/1
  Rate Transition3/1 -> Observe out2/1
  Signal Specification/1 -> Rate Transition/1
  Rate Transition4/1 -> VREP_SIMULINK_SYS_OBJ/2
  Signal Specification1/1 -> Rate Transition4/1
  Control In1/1 -> Signal Specification1/1
  VREP_SIMULINK_SYS_OBJ/2 -> Rate Transition2/1
  VREP_SIMULINK_SYS_OBJ/4 -> Mux/1
  VREP_SIMULINK_SYS_OBJ/5 -> Mux/2
  VREP_SIMULINK_SYS_OBJ/6 -> Mux/3
  VREP_SIMULINK_SYS_OBJ/7 -> Mux/4
  VREP_SIMULINK_SYS_OBJ/8 -> Mux/5
  VREP_SIMULINK_SYS_OBJ/9 -> Mux/6
  Mux/1 -> Rate Transition5/1
  Rate Transition5/1 -> Product/1
  Product/1 -> Observe out3/1
  Constant/1 -> Product/2

== system EKF_SIL_02_newdelIps/EKF/Control Signal ==
  Constant : Constant  Value=0
  Gain : Gain  Gain=-.5
  Mux : Mux  Inputs=6
  Mux1 : Mux  Inputs=3
  Step : Step  Time=5  After=-0.1
  d_theta_l : Outport
  d_theta : Outport  Port=2
  wires:
  Mux/1 -> d_theta/1
  Mux1/1 -> d_theta_l/1
  Constant/1 -> Mux/6, Mux/5, Mux/4
  Gain/1 -> Mux1/2, Mux1/1, Mux/1, Mux/2
  Step/1 -> Mux/3, Mux1/3, Gain/1

== system EKF_SIL_02_newdelIps/EKF/Create Bus [State Vector,X_a]1 ==
  X : Inport
  Bus Creator{1,3..5} (4 alike) : BusCreator  Inputs=3
  Bus Creator2 : BusCreator
  Bus Creator6 : BusCreator  Inputs=6
  Bus Creator7 : BusCreator
  Demux1 : Demux  Outputs=20
  X_bus : Outport
  wires:
  Bus Creator7/1 -> Bus Creator6/6  "ieps"
  Bus Creator1/1 -> Bus Creator6/5  "rho_c"
  Demux1/20 -> Bus Creator7/4  "ieps_0"
  Demux1/19 -> Bus Creator7/3  "ieps_3"
  Demux1/18 -> Bus Creator7/2  "ieps_2"
  Demux1/17 -> Bus Creator7/1  "ieps_1"
  Demux1/16 -> Bus Creator1/3  "rho_c_z"
  Demux1/15 -> Bus Creator1/2  "rho_c_y"
  Demux1/14 -> Bus Creator1/1  "rho_c_x"
  Demux1/13 -> Bus Creator5/3  "r_z_dot"
  Demux1/12 -> Bus Creator5/2  "r_y_dot"
  Demux1/11 -> Bus Creator5/1  "r_x_dot"
  Demux1/10 -> Bus Creator4/3  "r_z"
  Demux1/9 -> Bus Creator4/2  "r_y"
  Demux1/8 -> Bus Creator4/1  "r_x"
  Demux1/7 -> Bus Creator3/3  "omega_z"
  Demux1/6 -> Bus Creator3/2  "omega_y"
  Demux1/5 -> Bus Creator3/1  "omega_x"
  Demux1/4 -> Bus Creator2/4  "q_est_0"
  Demux1/3 -> Bus Creator2/3  "q_est_3"
  Demux1/2 -> Bus Creator2/2  "q_est_2"
  Demux1/1 -> Bus Creator2/1  "q_est_1"
  X/1 -> Demux1/1
  Bus Creator6/1 -> X_bus/1
  Bus Creator5/1 -> Bus Creator6/4  "r_dot"
  Bus Creator4/1 -> Bus Creator6/3  "r"
  Bus Creator3/1 -> Bus Creator6/2  "omega"
  Bus Creator2/1 -> Bus Creator6/1  "q_est"

== system EKF_SIL_02_newdelIps/EKF/Create Jacobian [b//ee] ==
  theta : Inport
  Interpreted MATLAB Function : MATLABFcn  MATLABFcn=J_1
  Interpreted MATLAB Function1 : MATLABFcn  MATLABFcn=J_2
  Interpreted MATLAB Function2 : MATLABFcn  MATLABFcn=J_3
  Interpreted MATLAB Function3 : MATLABFcn  MATLABFcn=J_4
  Interpreted MATLAB Function4 : MATLABFcn  MATLABFcn=J_5
  Interpreted MATLAB Function5 : MATLABFcn  MATLABFcn=J_6
  Math Function : Math  Operator=transpose  SaturateOnIntegerOverflow=on
  Matrix Concatenate : Concatenate  NumInputs=6  Mode=Multidimensional array  ConcatenateDimension=2
  J : Outport
  wires:
  Matrix Concatenate/1 -> J/1
  Interpreted MATLAB Function2/1 -> Matrix Concatenate/3
  Interpreted MATLAB Function/1 -> Matrix Concatenate/1
  theta/1 -> Math Function/1
  Interpreted MATLAB Function3/1 -> Matrix Concatenate/4
  Interpreted MATLAB Function1/1 -> Matrix Concatenate/2
  Interpreted MATLAB Function5/1 -> Matrix Concatenate/6
  Interpreted MATLAB Function4/1 -> Matrix Concatenate/5
  Math Function/1 -> Interpreted MATLAB Function2/1, Interpreted MATLAB Function1/1, Interpreted MATLAB Function/1, Interpreted MATLAB Function5/1, Interpreted MATLAB Function4/1, Interpreted MATLAB Function3/1

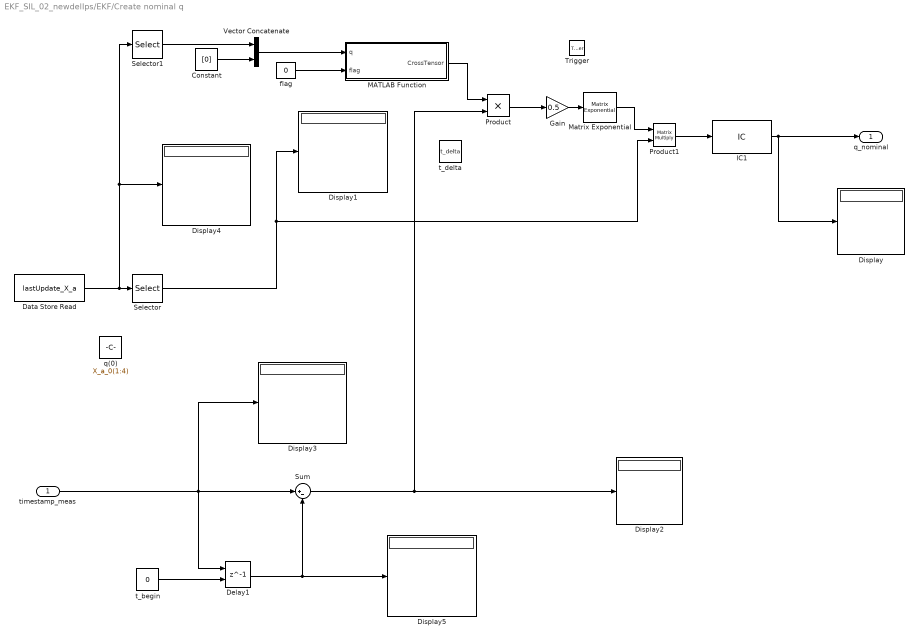
== system EKF_SIL_02_newdelIps/EKF/Create nominal q ==
  timestamp_meas : Inport
  Trigger : TriggerPort  PortDimensions=1
  Constant : Constant  Value=[0]
  Data Store Read : DataStoreRead  DialogController=Simulink.DDGSource  DataStoreName=lastUpdate_X_a  DataStoreElements=lastUpdate_X_a
  Delay1 : Delay  DelayLength=1  InitialConditionSource=Input port  InitialCondition=0
      settings: InputPortMap=u0,p4
  Display{,1..5} (6 alike) : Display
  Gain : Gain  Gain=0.5
  IC1 : InitialCondition  Value=X_a_0(1:4)
  MATLAB Function : MATLAB Function  TreatAsAtomicUnit=on
  Matrix Exponential : dspmtrx3/Matrix Exponential
  Product : Product
  Product1 : Product  Multiplication=Matrix(*)
  Selector : Selector  InputPortWidth=20  Indices=[1:4]
  Selector1 : Selector  InputPortWidth=20  Indices=[5:7]
  Sum : Sum  Inputs=|+-
  Vector Concatenate : Concatenate
  flag : Constant  Value=0
  q(0) : Constant  Value=X_a_0(1:4)
  t_begin : Constant  Value=0
  "t_delta " : Constant  Value=t_delta
  q_nominal : Outport
  wires:
  MATLAB Function/1(CrossTensor) -> Product/1
  Sum/1 -> Display2/1, Product/2
  Selector1/1 -> Vector Concatenate/1
  Constant/1 -> Vector Concatenate/2
  flag/1 -> MATLAB Function/2(flag)
  Product/1 -> Gain/1
  Vector Concatenate/1 -> MATLAB Function/1(q)
  Product1/1 -> IC1/1
  Gain/1 -> Matrix Exponential/1
  Matrix Exponential/1 -> Product1/1
  IC1/1 -> Display/1, q_nominal/1
  Selector/1 -> Product1/2, Display1/1
  Data Store Read/1 -> Display4/1, Selector1/1, Selector/1
  timestamp_meas/1 -> Display3/1, Delay1/1, Sum/1
  Delay1/1 -> Display5/1, Sum/2
  t_begin/1 -> Delay1/2

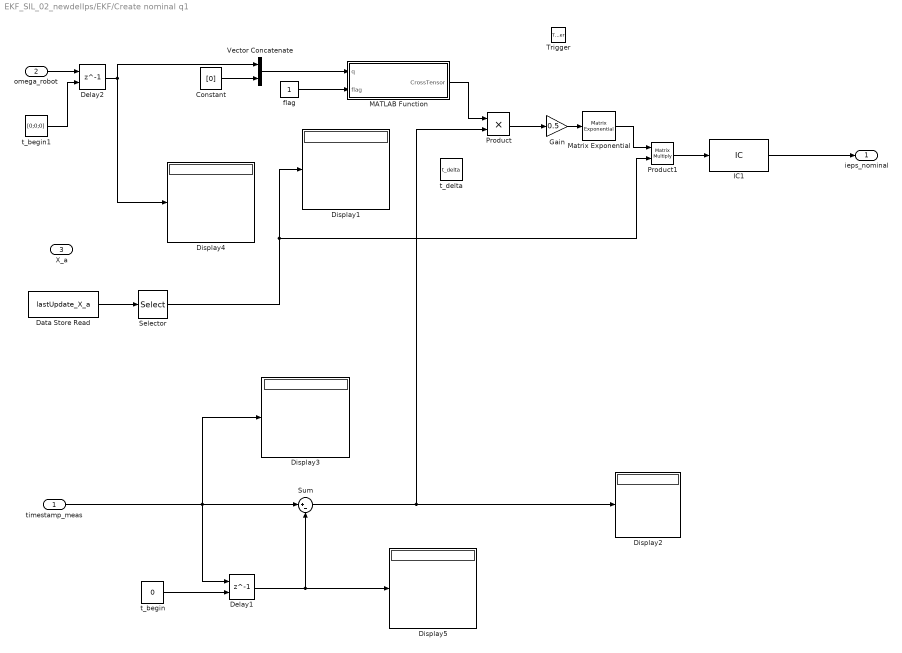
== system EKF_SIL_02_newdelIps/EKF/Create nominal q1 ==
  timestamp_meas : Inport
  omega_robot : Inport  Port=2
  X_a : Inport  Port=3
  Trigger : TriggerPort  PortDimensions=1
  Constant : Constant  Value=[0]
  Data Store Read : DataStoreRead  DialogController=Simulink.DDGSource  DataStoreName=lastUpdate_X_a  DataStoreElements=lastUpdate_X_a
  Delay1 : Delay  DelayLength=1  InitialConditionSource=Input port  InitialCondition=0
      settings: InputPortMap=u0,p4
  Delay2 : Delay  DelayLength=1  InitialConditionSource=Input port  InitialCondition=0
      settings: InputPortMap=u0,p4
  Display{1..5} (5 alike) : Display
  Gain : Gain  Gain=0.5
  IC1 : InitialCondition  Value=X_a_0(17:20)
  MATLAB Function : MATLAB Function  TreatAsAtomicUnit=on
  Matrix Exponential : dspmtrx3/Matrix Exponential
  Product : Product
  Product1 : Product  Multiplication=Matrix(*)
  Selector : Selector  InputPortWidth=20  Indices=[17:20]
  Sum : Sum  Inputs=|+-
  Vector Concatenate : Concatenate
  flag : Constant
  t_begin : Constant  Value=0
  t_begin1 : Constant  Value=[0;0;0]
  "t_delta " : Constant  Value=t_delta
  ieps_nominal : Outport
  wires:
  t_begin/1 -> Delay1/2
  Delay1/1 -> Sum/2, Display5/1
  timestamp_meas/1 -> Sum/1, Delay1/1, Display3/1
  Selector/1 -> Display1/1, Product1/2
  IC1/1 -> ieps_nominal/1
  Matrix Exponential/1 -> Product1/1
  Gain/1 -> Matrix Exponential/1
  Product1/1 -> IC1/1
  Vector Concatenate/1 -> MATLAB Function/1(q)
  Product/1 -> Gain/1
  flag/1 -> MATLAB Function/2(flag)
  Constant/1 -> Vector Concatenate/2
  Delay2/1 -> Vector Concatenate/1, Display4/1
  Sum/1 -> Product/2, Display2/1
  MATLAB Function/1(CrossTensor) -> Product/1
  Data Store Read/1 -> Selector/1
  omega_robot/1 -> Delay2/1
  t_begin1/1 -> Delay2/2

== system EKF_SIL_02_newdelIps/EKF/Initial Conditions (create bus) ==
  Bus Creator : BusCreator
  Bus Creator{1..3,5} (4 alike) : BusCreator  Inputs=3
  Bus Creator4 : BusCreator  Inputs=6
  Bus Creator6 : BusCreator
  Demux : Demux  Outputs=20
  Initial conditions (null vector) : Constant  Value=[X_a_0]
  Initial conditions (known) : FromFile  FileName=X_a_0_Model_02.mat
  P_post : Constant  Value=P_0  VectorParams1D=off
  "X_a(0) " : Outport
  "P_post " : Outport  Port=2
  wires:
  Demux/1 -> Bus Creator/1  "q_1"
  Demux/2 -> Bus Creator/2  "q_2"
  Demux/3 -> Bus Creator/3  "q_3"
  Demux/4 -> Bus Creator/4  "q_0"
  Demux/5 -> Bus Creator1/1  "omega_x"
  Demux/6 -> Bus Creator1/2  "omega_y"
  Demux/7 -> Bus Creator1/3  "omega_z"
  Demux/8 -> Bus Creator2/1  "r_x"
  Demux/9 -> Bus Creator2/2  "r_y"
  Demux/10 -> Bus Creator2/3  "r_z"
  Demux/11 -> Bus Creator3/1  "r_x_dot"
  Demux/12 -> Bus Creator3/2  "r_y_dot"
  Demux/13 -> Bus Creator3/3  "r_z_dot"
  Bus Creator/1 -> Bus Creator4/1  "q_est"
  Bus Creator1/1 -> Bus Creator4/2  "omega"
  Bus Creator2/1 -> Bus Creator4/3  "r"
  Bus Creator3/1 -> Bus Creator4/4  "r_dot"
  Bus Creator4/1 -> "X_a(0) "/1  "X_a(0)"
  P_post/1 -> "P_post "/1
  Initial conditions (null vector)/1 -> Demux/1
  Demux/14 -> Bus Creator5/1  "rho_c_x"
  Demux/15 -> Bus Creator5/2  "rho_c_y"
  Demux/16 -> Bus Creator5/3  "rho_c_z"
  Demux/17 -> Bus Creator6/1  "ieps_1"
  Demux/18 -> Bus Creator6/2  "ieps_2"
  Demux/19 -> Bus Creator6/3  "ieps_3"
  Demux/20 -> Bus Creator6/4  "ieps_0"
  Bus Creator5/1 -> Bus Creator4/5  "rho_c"
  Bus Creator6/1 -> Bus Creator4/6  "ieps"

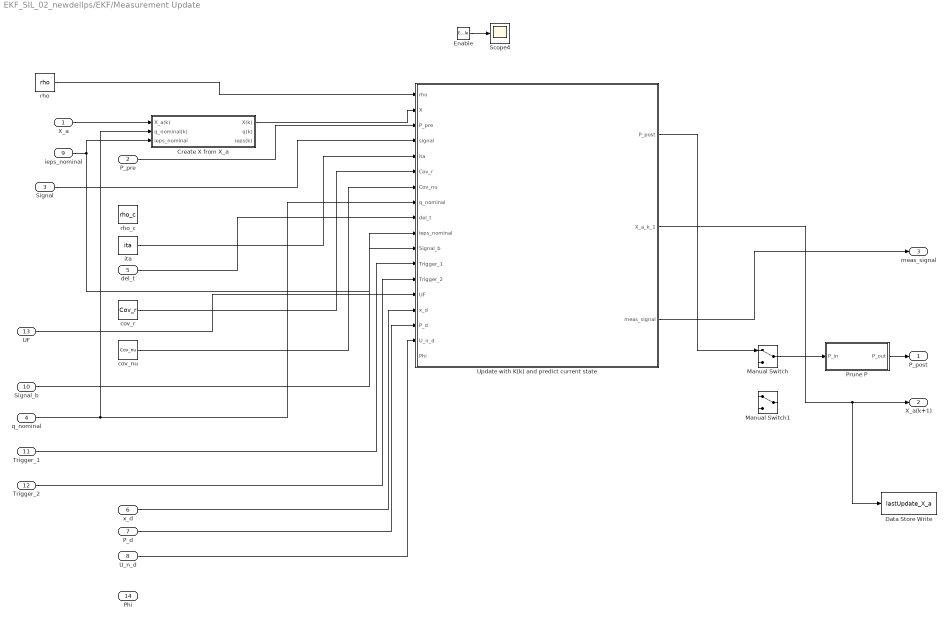
== system EKF_SIL_02_newdelIps/EKF/Measurement Update ==
  X_a : Inport
  P_pre : Inport  Port=2
  Signal : Inport  Port=3
  "q_nominal " : Inport  Port=4
  del_t : Inport  Port=5
  x_d : Inport  Port=6
  P_d : Inport  Port=7
  U_n_d : Inport  Port=8
  ieps_nominal : Inport  Port=9
  Signal_b : Inport  Port=10
  Trigger_1 : Inport  Port=11
  Trigger_2 : Inport  Port=12
  UF : Inport  Port=13
  Phi : Inport  Port=14
  Enable : EnablePort  PropagateVarSize=During execution  ShowOutputPort=on
  Create X from X_a : Subsystem
  Data Store Write : DataStoreWrite  DialogController=Simulink.DDGSource  DataStoreName=lastUpdate_X_a
  Manual Switch : ManualSwitch
  Manual Switch1 : ManualSwitch
  Prune P : Subsystem
  Scope4 : Scope
      settings: YMin=0  YMax=1  SaveName=ScopeData27
  Update with K(k) and predict current state : Subsystem
  cov_nu : Constant  Value=Cov_nu
  cov_r : Constant  Value=Cov_r
  "ita " : Constant  Value=ita
  "rho " : Constant  Value=rho
  rho_c : Constant  Value=rho_c
  P_post : Outport
  X_a(k+1) : Outport  Port=2
  meas_signal : Outport  Port=3
  wires:
  "ita "/1 -> Update with K(k) and predict current state/5(ita)
  cov_r/1 -> Update with K(k) and predict current state/6(Cov_r)
  cov_nu/1 -> Update with K(k) and predict current state/7(Cov_nu)
  Enable/1 -> Scope4/1
  del_t/1 -> Update with K(k) and predict current state/9(del_t)
  "q_nominal "/1 -> Create X from X_a/2(q_nominal(k)), Update with K(k) and predict current state/8(q_nominal)
  "rho "/1 -> Update with K(k) and predict current state/1(rho)
  Update with K(k) and predict current state/1(P_post) -> Manual Switch/1
  Create X from X_a/1(X(k)) -> Update with K(k) and predict current state/2(X)
  X_a/1 -> Create X from X_a/1(X_a(k))
  P_pre/1 -> Update with K(k) and predict current state/3(P_pre)
  Manual Switch/1 -> Prune P/1(P_in)
  Signal/1 -> Update with K(k) and predict current state/4(signal)
  Update with K(k) and predict current state/3(meas_signal) -> meas_signal/1
  Prune P/1(P_out) -> P_post/1
  ieps_nominal/1 -> Update with K(k) and predict current state/10(ieps_nominal), Create X from X_a/3(ieps_nominal)
  Update with K(k) and predict current state/2(X_a_k_1) -> X_a(k+1)/1, Data Store Write/1
  Signal_b/1 -> Update with K(k) and predict current state/11(Signal_b)
  Trigger_1/1 -> Update with K(k) and predict current state/12(Trigger_1)
  Trigger_2/1 -> Update with K(k) and predict current state/13(Trigger_2)
  UF/1 -> Update with K(k) and predict current state/14(UF)
  x_d/1 -> Update with K(k) and predict current state/15(x_d)
  P_d/1 -> Update with K(k) and predict current state/16(P_d)
  U_n_d/1 -> Update with K(k) and predict current state/17(U_n_d)

== system EKF_SIL_02_newdelIps/EKF/Predictor ==
  X_a(K) : Inport
  P_previous(k) : Inport  Port=2
  trigger : Inport  Port=3
  V : Inport  Port=4
  Create Bus [State Vector,X_a] : Subsystem
  Create Bus [State Vector,X_a]1 : Subsystem
  Create State error covariance (P) : Subsystem
  Delay : Delay  DelayLength=1  InitialCondition=0
  Dynamic Model (Differential equations)2 : Subsystem
  Product : Product
  Sum : Sum  Inputs=|++
  t_Kalman : Constant  Value=t_Kalman
  X_a(k+1) : Outport
  P_current(k+1) : Outport  Port=2
  wires:
  Create Bus [State Vector,X_a]1/1(X_bus) -> Create State error covariance (P)/1(X_a)
  Create State error covariance (P)/1(P_current) -> P_current(k+1)/1
  Dynamic Model (Differential equations)2/1(X_a_dot) -> Product/1
  P_previous(k)/1 -> Create State error covariance (P)/2(P_previous)
  trigger/1 -> Delay/1
  V/1 -> Create State error covariance (P)/3(V), Dynamic Model (Differential equations)2/2("V ")
  X_a(K)/1 -> Sum/2, Create Bus [State Vector,X_a]1/1(X), Dynamic Model (Differential equations)2/1(X_a(t))
  Create Bus [State Vector,X_a]/1(X_bus) -> X_a(k+1)/1
  t_Kalman/1 -> Product/2
  Product/1 -> Sum/1
  Sum/1 -> Create Bus [State Vector,X_a]/1(X)

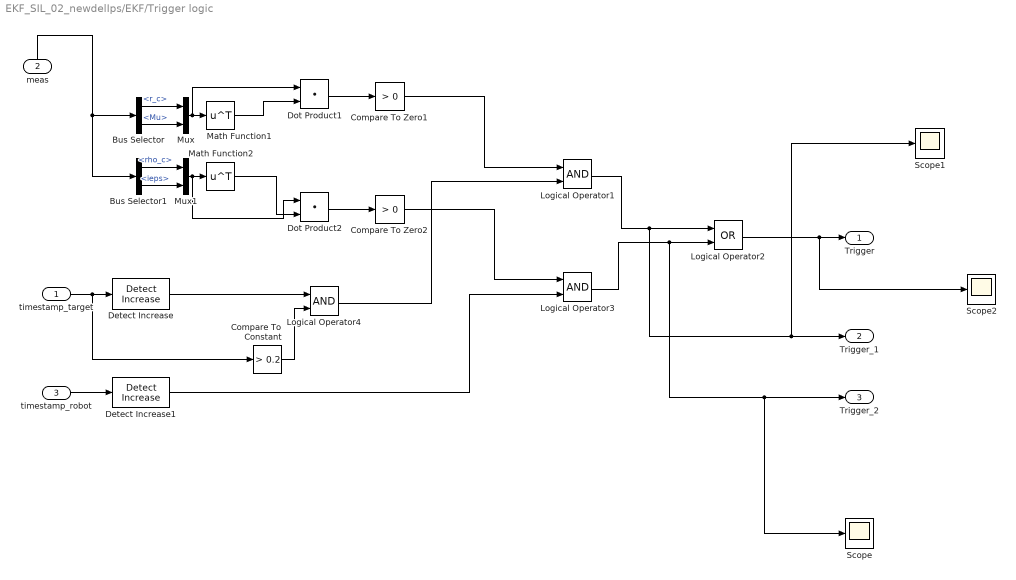
== system EKF_SIL_02_newdelIps/EKF/Trigger logic ==
  timestamp_target : Inport
  meas : Inport  Port=2
  timestamp_robot : Inport  Port=3
  Bus Selector : BusSelector  OutputSignals=r_c,Mu
  Bus Selector1 : BusSelector  OutputSignals=rho_c,ieps
  Compare To Constant : simulink/Logic and Bit Operations/Compare To Constant  relop=>  const=0.2  OutDataTypeStr=boolean
  Compare To Zero1 : simulink/Logic and Bit Operations/Compare To Zero  relop=>  OutDataTypeStr=boolean
  Compare To Zero2 : simulink/Logic and Bit Operations/Compare To Zero  relop=>  OutDataTypeStr=boolean
  Detect Increase : simulink/Logic and Bit Operations/Detect Increase  vinit=0  InputProcessing=Inherited  OutDataTypeStr=boolean
  Detect Increase1 : simulink/Logic and Bit Operations/Detect Increase  vinit=0  InputProcessing=Inherited  OutDataTypeStr=boolean
  Dot Product1 : DotProduct  InputSameDT=on  OutDataTypeStr=Inherit: Inherit via internal rule
  Dot Product2 : DotProduct  InputSameDT=on  OutDataTypeStr=Inherit: Inherit via internal rule
  Logical Operator1 : Logic  AllPortsSameDT=off  OutDataTypeStr=boolean
  Logical Operator2 : Logic  Operator=OR  AllPortsSameDT=off  OutDataTypeStr=boolean
  Logical Operator3 : Logic  AllPortsSameDT=off  OutDataTypeStr=boolean
  Logical Operator4 : Logic  AllPortsSameDT=off  OutDataTypeStr=boolean
  Math Function1 : Math  Operator=transpose  SaturateOnIntegerOverflow=on
  Math Function2 : Math  Operator=transpose  SaturateOnIntegerOverflow=on
  Mux : Mux  Inputs=2
  Mux1 : Mux  Inputs=2
  Scope : Scope
      settings: SaveName=ScopeData12
  Scope1 : Scope
      settings: SaveName=ScopeData13
  Scope2 : Scope
      settings: SaveName=ScopeData16
  "Trigger " : Outport
  "Trigger_1 " : Outport  Port=2
  "Trigger_2 " : Outport  Port=3
  wires:
  Logical Operator2/1 -> Scope2/1, "Trigger "/1
  meas/1 -> Bus Selector1/1, Bus Selector/1
  timestamp_target/1 -> Detect Increase/1, Compare To Constant/1
  Bus Selector/1 -> Mux/1  "<r_c>"
  Bus Selector/2 -> Mux/2  "<Mu>"
  Bus Selector1/1 -> Mux1/1  "<rho_c>"
  Bus Selector1/2 -> Mux1/2  "<ieps>"
  Math Function1/1 -> Dot Product1/2
  Mux/1 -> Dot Product1/1, Math Function1/1
  Mux1/1 -> Dot Product2/1, Math Function2/1
  Math Function2/1 -> Dot Product2/2
  Dot Product1/1 -> Compare To Zero1/1
  Dot Product2/1 -> Compare To Zero2/1
  Compare To Zero1/1 -> Logical Operator1/1
  timestamp_robot/1 -> Detect Increase1/1
  Logical Operator4/1 -> Logical Operator1/2
  Detect Increase1/1 -> Logical Operator3/2
  Compare To Zero2/1 -> Logical Operator3/1
  Logical Operator1/1 -> Scope1/1, "Trigger_1 "/1, Logical Operator2/1
  Logical Operator3/1 -> Scope/1, "Trigger_2 "/1, Logical Operator2/2
  Detect Increase/1 -> Logical Operator4/1
  Compare To Constant/1 -> Logical Operator4/2

== system EKF_SIL_02_newdelIps/Plant/Dynamic Model (Differential equations) ==
  X_a(t) : Inport
  Bus Creator : BusCreator
  Constant : Constant  Value=[0]
  Constant1 : Constant  Value=zeros(3,1)
  "Orbital Dynamics " : Subsystem
  Quaternion Kinematics : Subsystem
  Rotational Dynamics : Subsystem
  Vector Concatenate : Concatenate
  n : Constant  Value=n
  omega : Selector  NumberOfDimensions=2  InputPortWidth=3  IndexOptions=Index vector (dialog),Index vector (dialog)  Indices=[5 6 7],1  OutputSizes=1,1
  p : Constant  Value=[p_x;p_y;p_z]
  parameter_gravitation : Constant  Value=parameter_gravitation
  q : Selector  NumberOfDimensions=2  InputPortWidth=3  IndexOptions=Index vector (dialog),Index vector (dialog)  Indices=[1 2 3 4],1  OutputSizes=1,1
  r : Selector  NumberOfDimensions=2  InputPortWidth=3  IndexOptions=Index vector (dialog),Index vector (dialog)  Indices=[8 9 10],1  OutputSizes=1,1
  r_dot : Selector  NumberOfDimensions=2  InputPortWidth=3  IndexOptions=Index vector (dialog),Index vector (dialog)  Indices=[11 12 13],1  OutputSizes=1,1
  X_a(t+1) : Outport
  wires:
  Constant/1 -> Vector Concatenate/2
  p/1 -> Rotational Dynamics/2(p)
  Vector Concatenate/1 -> Quaternion Kinematics/2(omega_rel)
  parameter_gravitation/1 -> "Orbital Dynamics "/2(Mu)
  n/1 -> "Orbital Dynamics "/3(n)
  Quaternion Kinematics/1(q_dot) -> Bus Creator/1  "q_dot"
  Rotational Dynamics/1(omega_dot) -> Bus Creator/2  "omega_dot"
  X_a(t)/1 -> q/1, omega/1, r_dot/1, r/1
  q/1 -> Quaternion Kinematics/1(q)
  omega/1 -> Rotational Dynamics/1(omega), Vector Concatenate/1
  r/1 -> "Orbital Dynamics "/1(r)
  r_dot/1 -> "Orbital Dynamics "/4("r_dot "), Bus Creator/3
  Bus Creator/1 -> X_a(t+1)/1
  Constant1/1 -> Bus Creator/4

== system EKF_SIL_02_newdelIps/Plant/Initial Conditions (create bus) ==
  Bus Creator : BusCreator
  Bus Creator1 : BusCreator  Inputs=3
  Bus Creator2 : BusCreator  Inputs=3
  Bus Creator3 : BusCreator  Inputs=3
  Bus Creator4 : BusCreator
  Demux : Demux  Outputs=13
  Display : Display
  Initial conditions (Dynamic Model) : FromFile  FileName=X_a_0_Model_02.mat  SampleTime=0
  "X_a(0) " : Outport
  wires:
  Initial conditions (Dynamic Model)/1 -> Demux/1
  Demux/1 -> Bus Creator/1  "q_1"
  Demux/2 -> Bus Creator/2  "q_2"
  Demux/3 -> Bus Creator/3  "q_3"
  Demux/4 -> Bus Creator/4  "q_0"
  Demux/5 -> Bus Creator1/1  "omega_x"
  Demux/6 -> Bus Creator1/2  "omega_y"
  Demux/7 -> Bus Creator1/3  "omega_z"
  Demux/8 -> Bus Creator2/1  "r_x"
  Demux/9 -> Bus Creator2/2  "r_y"
  Demux/10 -> Bus Creator2/3  "r_z"
  Demux/11 -> Bus Creator3/1  "r_x_dot"
  Demux/12 -> Bus Creator3/2  "r_y_dot"
  Demux/13 -> Bus Creator3/3  "r_z_dot"
  Bus Creator/1 -> Bus Creator4/1  "q"
  Bus Creator1/1 -> Bus Creator4/2  "omega"
  Bus Creator2/1 -> Bus Creator4/3  "r"
  Bus Creator3/1 -> Bus Creator4/4  "r_dot"
  Bus Creator4/1 -> Display/1, "X_a(0) "/1  "X_a(0)"

== system EKF_SIL_02_newdelIps/Plots and display/Create Measurements [Pose]1 ==
  q : Inport
  r : Inport  Port=2
  rho : Inport  Port=3
  ita : Inport  Port=4
  "rho_c " : Inport  Port=5
  "Create Measurements [Orientation] " : Subsystem
  Create Measurements [Position] : Subsystem
  Rate Transition : RateTransition
  Rate Transition1 : RateTransition
  Rate Transition2 : RateTransition
  r_c : Outport
  Mu : Outport  Port=2
  wires:
  q/1 -> "Create Measurements [Orientation] "/1(q), Create Measurements [Position]/2(q)
  r/1 -> Create Measurements [Position]/1(r)
  "Create Measurements [Orientation] "/1(Mu) -> Mu/1
  ita/1 -> Rate Transition1/1
  Create Measurements [Position]/1(r_c) -> r_c/1
  rho/1 -> Rate Transition2/1
  "rho_c "/1 -> Rate Transition/1
  Rate Transition/1 -> Create Measurements [Position]/4("rho_c ")
  Rate Transition1/1 -> "Create Measurements [Orientation] "/2("ita ")
  Rate Transition2/1 -> Create Measurements [Position]/3(rho)

== system EKF_SIL_02_newdelIps/Plots and display/Create Measurements [Pose]2 ==
  q : Inport
  r : Inport  Port=2
  rho : Inport  Port=3
  ita : Inport  Port=4
  "rho_c " : Inport  Port=5
  ieps : Inport  Port=6
  "Create Measurements [Orientation] " : Subsystem
  Create Measurements [Position] : Subsystem
  Rate Transition : RateTransition
  Rate Transition1 : RateTransition
  Rate Transition2 : RateTransition
  r_c : Outport
  Mu : Outport  Port=2
  wires:
  Rate Transition2/1 -> Create Measurements [Position]/3(rho)
  Rate Transition1/1 -> "Create Measurements [Orientation] "/2("ita ")
  "rho_c "/1 -> Rate Transition/1
  rho/1 -> Rate Transition2/1
  Create Measurements [Position]/1(r_c) -> r_c/1
  ita/1 -> Rate Transition1/1
  "Create Measurements [Orientation] "/1(Mu) -> Mu/1
  r/1 -> Create Measurements [Position]/1(r)
  q/1 -> Create Measurements [Position]/2(q), "Create Measurements [Orientation] "/1(q)
  Rate Transition/1 -> Create Measurements [Position]/4("rho_c ")
  ieps/1 -> Create Measurements [Position]/5("ieps "), "Create Measurements [Orientation] "/3("ieps ")
